simulink model "carry_skip_adder"  (R2022b)
settings: Solver=FixedStepDiscrete  StartTime=0.0  StopTime=10.0  RelTol=1e-3
PreLoadFcn:
  | addpath('C:\Course_Material\UofT\ECE1718\assignment2\matlab_tests\hdlimport\carry_skip_adder');
libraries: simulink x240, hdlsllib x97
(part 2 of 2)

== system carry_skip_adder/carry_skip_adder/adder_4bit/full_adder03 ==
  a : Inport  OutDataTypeStr=fixdt(0, 1, 0)  SampleTime=-1
  b : Inport  Port=2  OutDataTypeStr=fixdt(0, 1, 0)  SampleTime=-1
  c_in : Inport  Port=3  OutDataTypeStr=fixdt(0, 1, 0)  SampleTime=-1
  Bit_AND : simulink/Logic and Bit Operations/Bitwise Operator  logicop=AND  UseBitMask=off  NumInputPorts=2  BitMask=double(0)  BitMaskRealWorld=Real World Value
  Bit_AND_1 : simulink/Logic and Bit Operations/Bitwise Operator  logicop=AND  UseBitMask=off  NumInputPorts=2  BitMask=double(0)  BitMaskRealWorld=Real World Value
  Bit_OR : simulink/Logic and Bit Operations/Bitwise Operator  logicop=OR  UseBitMask=off  NumInputPorts=2  BitMask=double(0)  BitMaskRealWorld=Real World Value
  Bit_XOR : simulink/Logic and Bit Operations/Bitwise Operator  logicop=XOR  UseBitMask=off  NumInputPorts=2  BitMask=double(0)  BitMaskRealWorld=Real World Value
  Bit_XOR_1 : simulink/Logic and Bit Operations/Bitwise Operator  logicop=XOR  UseBitMask=off  NumInputPorts=2  BitMask=double(0)  BitMaskRealWorld=Real World Value
  Bit_XOR_2 : simulink/Logic and Bit Operations/Bitwise Operator  logicop=XOR  UseBitMask=off  NumInputPorts=2  BitMask=double(0)  BitMaskRealWorld=Real World Value
  sum : Outport  OutDataTypeStr=fixdt(0, 1, 0)  SampleTime=-1
  c_out : Outport  Port=2  OutDataTypeStr=fixdt(0, 1, 0)  SampleTime=-1
  wires:
  a/1 -> Bit_AND_1/1, Bit_XOR_2/1, Bit_XOR_1/1
  b/1 -> Bit_AND_1/2, Bit_XOR_2/2, Bit_XOR_1/2
  Bit_AND/1 -> Bit_OR/1
  Bit_XOR/1 -> sum/1
  Bit_AND_1/1 -> Bit_OR/2
  Bit_XOR_2/1 -> Bit_AND/1
  Bit_XOR_1/1 -> Bit_XOR/1
  c_in/1 -> Bit_AND/2, Bit_XOR/2
  Bit_OR/1 -> c_out/1

== system carry_skip_adder/carry_skip_adder/adder_4bit1/full_adder0 ==
  a : Inport  OutDataTypeStr=fixdt(0, 1, 0)  SampleTime=-1
  b : Inport  Port=2  OutDataTypeStr=fixdt(0, 1, 0)  SampleTime=-1
  c_in : Inport  Port=3  OutDataTypeStr=fixdt(0, 1, 0)  SampleTime=-1
  Bit_AND : simulink/Logic and Bit Operations/Bitwise Operator  logicop=AND  UseBitMask=off  NumInputPorts=2  BitMask=double(0)  BitMaskRealWorld=Real World Value
  Bit_AND_1 : simulink/Logic and Bit Operations/Bitwise Operator  logicop=AND  UseBitMask=off  NumInputPorts=2  BitMask=double(0)  BitMaskRealWorld=Real World Value
  Bit_OR : simulink/Logic and Bit Operations/Bitwise Operator  logicop=OR  UseBitMask=off  NumInputPorts=2  BitMask=double(0)  BitMaskRealWorld=Real World Value
  Bit_XOR : simulink/Logic and Bit Operations/Bitwise Operator  logicop=XOR  UseBitMask=off  NumInputPorts=2  BitMask=double(0)  BitMaskRealWorld=Real World Value
  Bit_XOR_1 : simulink/Logic and Bit Operations/Bitwise Operator  logicop=XOR  UseBitMask=off  NumInputPorts=2  BitMask=double(0)  BitMaskRealWorld=Real World Value
  Bit_XOR_2 : simulink/Logic and Bit Operations/Bitwise Operator  logicop=XOR  UseBitMask=off  NumInputPorts=2  BitMask=double(0)  BitMaskRealWorld=Real World Value
  sum : Outport  OutDataTypeStr=fixdt(0, 1, 0)  SampleTime=-1
  c_out : Outport  Port=2  OutDataTypeStr=fixdt(0, 1, 0)  SampleTime=-1
  wires:
  a/1 -> Bit_AND_1/1, Bit_XOR_2/1, Bit_XOR_1/1
  Bit_XOR_1/1 -> Bit_XOR/1
  b/1 -> Bit_AND_1/2, Bit_XOR_2/2, Bit_XOR_1/2
  c_in/1 -> Bit_AND/2, Bit_XOR/2
  Bit_XOR/1 -> sum/1
  Bit_AND_1/1 -> Bit_OR/2
  Bit_XOR_2/1 -> Bit_AND/1
  Bit_AND/1 -> Bit_OR/1
  Bit_OR/1 -> c_out/1

== system carry_skip_adder/carry_skip_adder/adder_4bit1/full_adder01 ==
  a : Inport  OutDataTypeStr=fixdt(0, 1, 0)  SampleTime=-1
  b : Inport  Port=2  OutDataTypeStr=fixdt(0, 1, 0)  SampleTime=-1
  c_in : Inport  Port=3  OutDataTypeStr=fixdt(0, 1, 0)  SampleTime=-1
  Bit_AND : simulink/Logic and Bit Operations/Bitwise Operator  logicop=AND  UseBitMask=off  NumInputPorts=2  BitMask=double(0)  BitMaskRealWorld=Real World Value
  Bit_AND_1 : simulink/Logic and Bit Operations/Bitwise Operator  logicop=AND  UseBitMask=off  NumInputPorts=2  BitMask=double(0)  BitMaskRealWorld=Real World Value
  Bit_OR : simulink/Logic and Bit Operations/Bitwise Operator  logicop=OR  UseBitMask=off  NumInputPorts=2  BitMask=double(0)  BitMaskRealWorld=Real World Value
  Bit_XOR : simulink/Logic and Bit Operations/Bitwise Operator  logicop=XOR  UseBitMask=off  NumInputPorts=2  BitMask=double(0)  BitMaskRealWorld=Real World Value
  Bit_XOR_1 : simulink/Logic and Bit Operations/Bitwise Operator  logicop=XOR  UseBitMask=off  NumInputPorts=2  BitMask=double(0)  BitMaskRealWorld=Real World Value
  Bit_XOR_2 : simulink/Logic and Bit Operations/Bitwise Operator  logicop=XOR  UseBitMask=off  NumInputPorts=2  BitMask=double(0)  BitMaskRealWorld=Real World Value
  sum : Outport  OutDataTypeStr=fixdt(0, 1, 0)  SampleTime=-1
  c_out : Outport  Port=2  OutDataTypeStr=fixdt(0, 1, 0)  SampleTime=-1
  wires:
  a/1 -> Bit_AND_1/1, Bit_XOR_2/1, Bit_XOR_1/1
  Bit_AND/1 -> Bit_OR/1
  b/1 -> Bit_AND_1/2, Bit_XOR_1/2, Bit_XOR_2/2
  Bit_AND_1/1 -> Bit_OR/2
  Bit_XOR_1/1 -> Bit_XOR/1
  c_in/1 -> Bit_AND/2, Bit_XOR/2
  Bit_XOR/1 -> sum/1
  Bit_XOR_2/1 -> Bit_AND/1
  Bit_OR/1 -> c_out/1

== system carry_skip_adder/carry_skip_adder/adder_4bit1/full_adder02 ==
  a : Inport  OutDataTypeStr=fixdt(0, 1, 0)  SampleTime=-1
  b : Inport  Port=2  OutDataTypeStr=fixdt(0, 1, 0)  SampleTime=-1
  c_in : Inport  Port=3  OutDataTypeStr=fixdt(0, 1, 0)  SampleTime=-1
  Bit_AND : simulink/Logic and Bit Operations/Bitwise Operator  logicop=AND  UseBitMask=off  NumInputPorts=2  BitMask=double(0)  BitMaskRealWorld=Real World Value
  Bit_AND_1 : simulink/Logic and Bit Operations/Bitwise Operator  logicop=AND  UseBitMask=off  NumInputPorts=2  BitMask=double(0)  BitMaskRealWorld=Real World Value
  Bit_OR : simulink/Logic and Bit Operations/Bitwise Operator  logicop=OR  UseBitMask=off  NumInputPorts=2  BitMask=double(0)  BitMaskRealWorld=Real World Value
  Bit_XOR : simulink/Logic and Bit Operations/Bitwise Operator  logicop=XOR  UseBitMask=off  NumInputPorts=2  BitMask=double(0)  BitMaskRealWorld=Real World Value
  Bit_XOR_1 : simulink/Logic and Bit Operations/Bitwise Operator  logicop=XOR  UseBitMask=off  NumInputPorts=2  BitMask=double(0)  BitMaskRealWorld=Real World Value
  Bit_XOR_2 : simulink/Logic and Bit Operations/Bitwise Operator  logicop=XOR  UseBitMask=off  NumInputPorts=2  BitMask=double(0)  BitMaskRealWorld=Real World Value
  sum : Outport  OutDataTypeStr=fixdt(0, 1, 0)  SampleTime=-1
  c_out : Outport  Port=2  OutDataTypeStr=fixdt(0, 1, 0)  SampleTime=-1
  wires:
  a/1 -> Bit_AND_1/1, Bit_XOR_2/1, Bit_XOR_1/1
  b/1 -> Bit_AND_1/2, Bit_XOR_2/2, Bit_XOR_1/2
  Bit_AND_1/1 -> Bit_OR/2
  Bit_XOR_1/1 -> Bit_XOR/1
  c_in/1 -> Bit_XOR/2, Bit_AND/2
  Bit_XOR/1 -> sum/1
  Bit_XOR_2/1 -> Bit_AND/1
  Bit_AND/1 -> Bit_OR/1
  Bit_OR/1 -> c_out/1

== system carry_skip_adder/carry_skip_adder/adder_4bit1/full_adder03 ==
  a : Inport  OutDataTypeStr=fixdt(0, 1, 0)  SampleTime=-1
  b : Inport  Port=2  OutDataTypeStr=fixdt(0, 1, 0)  SampleTime=-1
  c_in : Inport  Port=3  OutDataTypeStr=fixdt(0, 1, 0)  SampleTime=-1
  Bit_AND : simulink/Logic and Bit Operations/Bitwise Operator  logicop=AND  UseBitMask=off  NumInputPorts=2  BitMask=double(0)  BitMaskRealWorld=Real World Value
  Bit_AND_1 : simulink/Logic and Bit Operations/Bitwise Operator  logicop=AND  UseBitMask=off  NumInputPorts=2  BitMask=double(0)  BitMaskRealWorld=Real World Value
  Bit_OR : simulink/Logic and Bit Operations/Bitwise Operator  logicop=OR  UseBitMask=off  NumInputPorts=2  BitMask=double(0)  BitMaskRealWorld=Real World Value
  Bit_XOR : simulink/Logic and Bit Operations/Bitwise Operator  logicop=XOR  UseBitMask=off  NumInputPorts=2  BitMask=double(0)  BitMaskRealWorld=Real World Value
  Bit_XOR_1 : simulink/Logic and Bit Operations/Bitwise Operator  logicop=XOR  UseBitMask=off  NumInputPorts=2  BitMask=double(0)  BitMaskRealWorld=Real World Value
  Bit_XOR_2 : simulink/Logic and Bit Operations/Bitwise Operator  logicop=XOR  UseBitMask=off  NumInputPorts=2  BitMask=double(0)  BitMaskRealWorld=Real World Value
  sum : Outport  OutDataTypeStr=fixdt(0, 1, 0)  SampleTime=-1
  c_out : Outport  Port=2  OutDataTypeStr=fixdt(0, 1, 0)  SampleTime=-1
  wires:
  Bit_XOR/1 -> sum/1
  Bit_XOR_2/1 -> Bit_AND/1
  a/1 -> Bit_AND_1/1, Bit_XOR_2/1, Bit_XOR_1/1
  Bit_AND/1 -> Bit_OR/1
  Bit_AND_1/1 -> Bit_OR/2
  b/1 -> Bit_AND_1/2, Bit_XOR_2/2, Bit_XOR_1/2
  Bit_XOR_1/1 -> Bit_XOR/1
  c_in/1 -> Bit_AND/2, Bit_XOR/2
  Bit_OR/1 -> c_out/1

== system carry_skip_adder/carry_skip_adder/adder_4bit2/full_adder0 ==
  a : Inport  OutDataTypeStr=fixdt(0, 1, 0)  SampleTime=-1
  b : Inport  Port=2  OutDataTypeStr=fixdt(0, 1, 0)  SampleTime=-1
  c_in : Inport  Port=3  OutDataTypeStr=fixdt(0, 1, 0)  SampleTime=-1
  Bit_AND : simulink/Logic and Bit Operations/Bitwise Operator  logicop=AND  UseBitMask=off  NumInputPorts=2  BitMask=double(0)  BitMaskRealWorld=Real World Value
  Bit_AND_1 : simulink/Logic and Bit Operations/Bitwise Operator  logicop=AND  UseBitMask=off  NumInputPorts=2  BitMask=double(0)  BitMaskRealWorld=Real World Value
  Bit_OR : simulink/Logic and Bit Operations/Bitwise Operator  logicop=OR  UseBitMask=off  NumInputPorts=2  BitMask=double(0)  BitMaskRealWorld=Real World Value
  Bit_XOR : simulink/Logic and Bit Operations/Bitwise Operator  logicop=XOR  UseBitMask=off  NumInputPorts=2  BitMask=double(0)  BitMaskRealWorld=Real World Value
  Bit_XOR_1 : simulink/Logic and Bit Operations/Bitwise Operator  logicop=XOR  UseBitMask=off  NumInputPorts=2  BitMask=double(0)  BitMaskRealWorld=Real World Value
  Bit_XOR_2 : simulink/Logic and Bit Operations/Bitwise Operator  logicop=XOR  UseBitMask=off  NumInputPorts=2  BitMask=double(0)  BitMaskRealWorld=Real World Value
  sum : Outport  OutDataTypeStr=fixdt(0, 1, 0)  SampleTime=-1
  c_out : Outport  Port=2  OutDataTypeStr=fixdt(0, 1, 0)  SampleTime=-1
  wires:
  a/1 -> Bit_XOR_2/1, Bit_AND_1/1, Bit_XOR_1/1
  Bit_XOR_1/1 -> Bit_XOR/1
  b/1 -> Bit_XOR_2/2, Bit_AND_1/2, Bit_XOR_1/2
  Bit_XOR/1 -> sum/1
  c_in/1 -> Bit_AND/2, Bit_XOR/2
  Bit_XOR_2/1 -> Bit_AND/1
  Bit_AND_1/1 -> Bit_OR/2
  Bit_AND/1 -> Bit_OR/1
  Bit_OR/1 -> c_out/1

== system carry_skip_adder/carry_skip_adder/adder_4bit2/full_adder01 ==
  a : Inport  OutDataTypeStr=fixdt(0, 1, 0)  SampleTime=-1
  b : Inport  Port=2  OutDataTypeStr=fixdt(0, 1, 0)  SampleTime=-1
  c_in : Inport  Port=3  OutDataTypeStr=fixdt(0, 1, 0)  SampleTime=-1
  Bit_AND : simulink/Logic and Bit Operations/Bitwise Operator  logicop=AND  UseBitMask=off  NumInputPorts=2  BitMask=double(0)  BitMaskRealWorld=Real World Value
  Bit_AND_1 : simulink/Logic and Bit Operations/Bitwise Operator  logicop=AND  UseBitMask=off  NumInputPorts=2  BitMask=double(0)  BitMaskRealWorld=Real World Value
  Bit_OR : simulink/Logic and Bit Operations/Bitwise Operator  logicop=OR  UseBitMask=off  NumInputPorts=2  BitMask=double(0)  BitMaskRealWorld=Real World Value
  Bit_XOR : simulink/Logic and Bit Operations/Bitwise Operator  logicop=XOR  UseBitMask=off  NumInputPorts=2  BitMask=double(0)  BitMaskRealWorld=Real World Value
  Bit_XOR_1 : simulink/Logic and Bit Operations/Bitwise Operator  logicop=XOR  UseBitMask=off  NumInputPorts=2  BitMask=double(0)  BitMaskRealWorld=Real World Value
  Bit_XOR_2 : simulink/Logic and Bit Operations/Bitwise Operator  logicop=XOR  UseBitMask=off  NumInputPorts=2  BitMask=double(0)  BitMaskRealWorld=Real World Value
  sum : Outport  OutDataTypeStr=fixdt(0, 1, 0)  SampleTime=-1
  c_out : Outport  Port=2  OutDataTypeStr=fixdt(0, 1, 0)  SampleTime=-1
  wires:
  a/1 -> Bit_AND_1/1, Bit_XOR_2/1, Bit_XOR_1/1
  Bit_AND/1 -> Bit_OR/1
  b/1 -> Bit_XOR_2/2, Bit_XOR_1/2, Bit_AND_1/2
  Bit_AND_1/1 -> Bit_OR/2
  Bit_XOR_1/1 -> Bit_XOR/1
  c_in/1 -> Bit_AND/2, Bit_XOR/2
  Bit_XOR/1 -> sum/1
  Bit_XOR_2/1 -> Bit_AND/1
  Bit_OR/1 -> c_out/1

== system carry_skip_adder/carry_skip_adder/adder_4bit2/full_adder02 ==
  a : Inport  OutDataTypeStr=fixdt(0, 1, 0)  SampleTime=-1
  b : Inport  Port=2  OutDataTypeStr=fixdt(0, 1, 0)  SampleTime=-1
  c_in : Inport  Port=3  OutDataTypeStr=fixdt(0, 1, 0)  SampleTime=-1
  Bit_AND : simulink/Logic and Bit Operations/Bitwise Operator  logicop=AND  UseBitMask=off  NumInputPorts=2  BitMask=double(0)  BitMaskRealWorld=Real World Value
  Bit_AND_1 : simulink/Logic and Bit Operations/Bitwise Operator  logicop=AND  UseBitMask=off  NumInputPorts=2  BitMask=double(0)  BitMaskRealWorld=Real World Value
  Bit_OR : simulink/Logic and Bit Operations/Bitwise Operator  logicop=OR  UseBitMask=off  NumInputPorts=2  BitMask=double(0)  BitMaskRealWorld=Real World Value
  Bit_XOR : simulink/Logic and Bit Operations/Bitwise Operator  logicop=XOR  UseBitMask=off  NumInputPorts=2  BitMask=double(0)  BitMaskRealWorld=Real World Value
  Bit_XOR_1 : simulink/Logic and Bit Operations/Bitwise Operator  logicop=XOR  UseBitMask=off  NumInputPorts=2  BitMask=double(0)  BitMaskRealWorld=Real World Value
  Bit_XOR_2 : simulink/Logic and Bit Operations/Bitwise Operator  logicop=XOR  UseBitMask=off  NumInputPorts=2  BitMask=double(0)  BitMaskRealWorld=Real World Value
  sum : Outport  OutDataTypeStr=fixdt(0, 1, 0)  SampleTime=-1
  c_out : Outport  Port=2  OutDataTypeStr=fixdt(0, 1, 0)  SampleTime=-1
  wires:
  a/1 -> Bit_AND_1/1, Bit_XOR_2/1, Bit_XOR_1/1
  b/1 -> Bit_AND_1/2, Bit_XOR_2/2, Bit_XOR_1/2
  Bit_AND_1/1 -> Bit_OR/2
  Bit_XOR_1/1 -> Bit_XOR/1
  c_in/1 -> Bit_AND/2, Bit_XOR/2
  Bit_XOR/1 -> sum/1
  Bit_XOR_2/1 -> Bit_AND/1
  Bit_AND/1 -> Bit_OR/1
  Bit_OR/1 -> c_out/1

== system carry_skip_adder/carry_skip_adder/adder_4bit2/full_adder03 ==
  a : Inport  OutDataTypeStr=fixdt(0, 1, 0)  SampleTime=-1
  b : Inport  Port=2  OutDataTypeStr=fixdt(0, 1, 0)  SampleTime=-1
  c_in : Inport  Port=3  OutDataTypeStr=fixdt(0, 1, 0)  SampleTime=-1
  Bit_AND : simulink/Logic and Bit Operations/Bitwise Operator  logicop=AND  UseBitMask=off  NumInputPorts=2  BitMask=double(0)  BitMaskRealWorld=Real World Value
  Bit_AND_1 : simulink/Logic and Bit Operations/Bitwise Operator  logicop=AND  UseBitMask=off  NumInputPorts=2  BitMask=double(0)  BitMaskRealWorld=Real World Value
  Bit_OR : simulink/Logic and Bit Operations/Bitwise Operator  logicop=OR  UseBitMask=off  NumInputPorts=2  BitMask=double(0)  BitMaskRealWorld=Real World Value
  Bit_XOR : simulink/Logic and Bit Operations/Bitwise Operator  logicop=XOR  UseBitMask=off  NumInputPorts=2  BitMask=double(0)  BitMaskRealWorld=Real World Value
  Bit_XOR_1 : simulink/Logic and Bit Operations/Bitwise Operator  logicop=XOR  UseBitMask=off  NumInputPorts=2  BitMask=double(0)  BitMaskRealWorld=Real World Value
  Bit_XOR_2 : simulink/Logic and Bit Operations/Bitwise Operator  logicop=XOR  UseBitMask=off  NumInputPorts=2  BitMask=double(0)  BitMaskRealWorld=Real World Value
  sum : Outport  OutDataTypeStr=fixdt(0, 1, 0)  SampleTime=-1
  c_out : Outport  Port=2  OutDataTypeStr=fixdt(0, 1, 0)  SampleTime=-1
  wires:
  a/1 -> Bit_AND_1/1, Bit_XOR_2/1, Bit_XOR_1/1
  Bit_AND/1 -> Bit_OR/1
  b/1 -> Bit_XOR_2/2, Bit_XOR_1/2, Bit_AND_1/2
  Bit_AND_1/1 -> Bit_OR/2
  Bit_XOR_1/1 -> Bit_XOR/1
  c_in/1 -> Bit_AND/2, Bit_XOR/2
  Bit_XOR/1 -> sum/1
  Bit_XOR_2/1 -> Bit_AND/1
  Bit_OR/1 -> c_out/1

== system carry_skip_adder/carry_skip_adder/adder_4bit3/full_adder0 ==
  a : Inport  OutDataTypeStr=fixdt(0, 1, 0)  SampleTime=-1
  b : Inport  Port=2  OutDataTypeStr=fixdt(0, 1, 0)  SampleTime=-1
  c_in : Inport  Port=3  OutDataTypeStr=fixdt(0, 1, 0)  SampleTime=-1
  Bit_AND : simulink/Logic and Bit Operations/Bitwise Operator  logicop=AND  UseBitMask=off  NumInputPorts=2  BitMask=double(0)  BitMaskRealWorld=Real World Value
  Bit_AND_1 : simulink/Logic and Bit Operations/Bitwise Operator  logicop=AND  UseBitMask=off  NumInputPorts=2  BitMask=double(0)  BitMaskRealWorld=Real World Value
  Bit_OR : simulink/Logic and Bit Operations/Bitwise Operator  logicop=OR  UseBitMask=off  NumInputPorts=2  BitMask=double(0)  BitMaskRealWorld=Real World Value
  Bit_XOR : simulink/Logic and Bit Operations/Bitwise Operator  logicop=XOR  UseBitMask=off  NumInputPorts=2  BitMask=double(0)  BitMaskRealWorld=Real World Value
  Bit_XOR_1 : simulink/Logic and Bit Operations/Bitwise Operator  logicop=XOR  UseBitMask=off  NumInputPorts=2  BitMask=double(0)  BitMaskRealWorld=Real World Value
  Bit_XOR_2 : simulink/Logic and Bit Operations/Bitwise Operator  logicop=XOR  UseBitMask=off  NumInputPorts=2  BitMask=double(0)  BitMaskRealWorld=Real World Value
  sum : Outport  OutDataTypeStr=fixdt(0, 1, 0)  SampleTime=-1
  c_out : Outport  Port=2  OutDataTypeStr=fixdt(0, 1, 0)  SampleTime=-1
  wires:
  Bit_AND_1/1 -> Bit_OR/2
  a/1 -> Bit_AND_1/1, Bit_XOR_2/1, Bit_XOR_1/1
  Bit_XOR_1/1 -> Bit_XOR/1
  b/1 -> Bit_AND_1/2, Bit_XOR_2/2, Bit_XOR_1/2
  c_in/1 -> Bit_AND/2, Bit_XOR/2
  Bit_XOR/1 -> sum/1
  Bit_XOR_2/1 -> Bit_AND/1
  Bit_AND/1 -> Bit_OR/1
  Bit_OR/1 -> c_out/1

== system carry_skip_adder/carry_skip_adder/adder_4bit3/full_adder01 ==
  a : Inport  OutDataTypeStr=fixdt(0, 1, 0)  SampleTime=-1
  b : Inport  Port=2  OutDataTypeStr=fixdt(0, 1, 0)  SampleTime=-1
  c_in : Inport  Port=3  OutDataTypeStr=fixdt(0, 1, 0)  SampleTime=-1
  Bit_AND : simulink/Logic and Bit Operations/Bitwise Operator  logicop=AND  UseBitMask=off  NumInputPorts=2  BitMask=double(0)  BitMaskRealWorld=Real World Value
  Bit_AND_1 : simulink/Logic and Bit Operations/Bitwise Operator  logicop=AND  UseBitMask=off  NumInputPorts=2  BitMask=double(0)  BitMaskRealWorld=Real World Value
  Bit_OR : simulink/Logic and Bit Operations/Bitwise Operator  logicop=OR  UseBitMask=off  NumInputPorts=2  BitMask=double(0)  BitMaskRealWorld=Real World Value
  Bit_XOR : simulink/Logic and Bit Operations/Bitwise Operator  logicop=XOR  UseBitMask=off  NumInputPorts=2  BitMask=double(0)  BitMaskRealWorld=Real World Value
  Bit_XOR_1 : simulink/Logic and Bit Operations/Bitwise Operator  logicop=XOR  UseBitMask=off  NumInputPorts=2  BitMask=double(0)  BitMaskRealWorld=Real World Value
  Bit_XOR_2 : simulink/Logic and Bit Operations/Bitwise Operator  logicop=XOR  UseBitMask=off  NumInputPorts=2  BitMask=double(0)  BitMaskRealWorld=Real World Value
  sum : Outport  OutDataTypeStr=fixdt(0, 1, 0)  SampleTime=-1
  c_out : Outport  Port=2  OutDataTypeStr=fixdt(0, 1, 0)  SampleTime=-1
  wires:
  a/1 -> Bit_AND_1/1, Bit_XOR_1/1, Bit_XOR_2/1
  Bit_AND/1 -> Bit_OR/1
  b/1 -> Bit_AND_1/2, Bit_XOR_2/2, Bit_XOR_1/2
  Bit_AND_1/1 -> Bit_OR/2
  Bit_XOR_1/1 -> Bit_XOR/1
  c_in/1 -> Bit_AND/2, Bit_XOR/2
  Bit_XOR/1 -> sum/1
  Bit_XOR_2/1 -> Bit_AND/1
  Bit_OR/1 -> c_out/1

== system carry_skip_adder/carry_skip_adder/adder_4bit3/full_adder02 ==
  a : Inport  OutDataTypeStr=fixdt(0, 1, 0)  SampleTime=-1
  b : Inport  Port=2  OutDataTypeStr=fixdt(0, 1, 0)  SampleTime=-1
  c_in : Inport  Port=3  OutDataTypeStr=fixdt(0, 1, 0)  SampleTime=-1
  Bit_AND : simulink/Logic and Bit Operations/Bitwise Operator  logicop=AND  UseBitMask=off  NumInputPorts=2  BitMask=double(0)  BitMaskRealWorld=Real World Value
  Bit_AND_1 : simulink/Logic and Bit Operations/Bitwise Operator  logicop=AND  UseBitMask=off  NumInputPorts=2  BitMask=double(0)  BitMaskRealWorld=Real World Value
  Bit_OR : simulink/Logic and Bit Operations/Bitwise Operator  logicop=OR  UseBitMask=off  NumInputPorts=2  BitMask=double(0)  BitMaskRealWorld=Real World Value
  Bit_XOR : simulink/Logic and Bit Operations/Bitwise Operator  logicop=XOR  UseBitMask=off  NumInputPorts=2  BitMask=double(0)  BitMaskRealWorld=Real World Value
  Bit_XOR_1 : simulink/Logic and Bit Operations/Bitwise Operator  logicop=XOR  UseBitMask=off  NumInputPorts=2  BitMask=double(0)  BitMaskRealWorld=Real World Value
  Bit_XOR_2 : simulink/Logic and Bit Operations/Bitwise Operator  logicop=XOR  UseBitMask=off  NumInputPorts=2  BitMask=double(0)  BitMaskRealWorld=Real World Value
  sum : Outport  OutDataTypeStr=fixdt(0, 1, 0)  SampleTime=-1
  c_out : Outport  Port=2  OutDataTypeStr=fixdt(0, 1, 0)  SampleTime=-1
  wires:
  a/1 -> Bit_AND_1/1, Bit_XOR_1/1, Bit_XOR_2/1
  b/1 -> Bit_AND_1/2, Bit_XOR_2/2, Bit_XOR_1/2
  Bit_AND_1/1 -> Bit_OR/2
  Bit_XOR_1/1 -> Bit_XOR/1
  c_in/1 -> Bit_AND/2, Bit_XOR/2
  Bit_XOR/1 -> sum/1
  Bit_XOR_2/1 -> Bit_AND/1
  Bit_AND/1 -> Bit_OR/1
  Bit_OR/1 -> c_out/1

== system carry_skip_adder/carry_skip_adder/adder_4bit3/full_adder03 ==
  a : Inport  OutDataTypeStr=fixdt(0, 1, 0)  SampleTime=-1
  b : Inport  Port=2  OutDataTypeStr=fixdt(0, 1, 0)  SampleTime=-1
  c_in : Inport  Port=3  OutDataTypeStr=fixdt(0, 1, 0)  SampleTime=-1
  Bit_AND : simulink/Logic and Bit Operations/Bitwise Operator  logicop=AND  UseBitMask=off  NumInputPorts=2  BitMask=double(0)  BitMaskRealWorld=Real World Value
  Bit_AND_1 : simulink/Logic and Bit Operations/Bitwise Operator  logicop=AND  UseBitMask=off  NumInputPorts=2  BitMask=double(0)  BitMaskRealWorld=Real World Value
  Bit_OR : simulink/Logic and Bit Operations/Bitwise Operator  logicop=OR  UseBitMask=off  NumInputPorts=2  BitMask=double(0)  BitMaskRealWorld=Real World Value
  Bit_XOR : simulink/Logic and Bit Operations/Bitwise Operator  logicop=XOR  UseBitMask=off  NumInputPorts=2  BitMask=double(0)  BitMaskRealWorld=Real World Value
  Bit_XOR_1 : simulink/Logic and Bit Operations/Bitwise Operator  logicop=XOR  UseBitMask=off  NumInputPorts=2  BitMask=double(0)  BitMaskRealWorld=Real World Value
  Bit_XOR_2 : simulink/Logic and Bit Operations/Bitwise Operator  logicop=XOR  UseBitMask=off  NumInputPorts=2  BitMask=double(0)  BitMaskRealWorld=Real World Value
  sum : Outport  OutDataTypeStr=fixdt(0, 1, 0)  SampleTime=-1
  c_out : Outport  Port=2  OutDataTypeStr=fixdt(0, 1, 0)  SampleTime=-1
  wires:
  a/1 -> Bit_AND_1/1, Bit_XOR_2/1, Bit_XOR_1/1
  Bit_AND/1 -> Bit_OR/1
  b/1 -> Bit_AND_1/2, Bit_XOR_1/2, Bit_XOR_2/2
  Bit_AND_1/1 -> Bit_OR/2
  Bit_XOR_1/1 -> Bit_XOR/1
  c_in/1 -> Bit_AND/2, Bit_XOR/2
  Bit_XOR/1 -> sum/1
  Bit_XOR_2/1 -> Bit_AND/1
  Bit_OR/1 -> c_out/1

== system carry_skip_adder/carry_skip_adder/adder_4bit4/full_adder0 ==
  a : Inport  OutDataTypeStr=fixdt(0, 1, 0)  SampleTime=-1
  b : Inport  Port=2  OutDataTypeStr=fixdt(0, 1, 0)  SampleTime=-1
  c_in : Inport  Port=3  OutDataTypeStr=fixdt(0, 1, 0)  SampleTime=-1
  Bit_AND : simulink/Logic and Bit Operations/Bitwise Operator  logicop=AND  UseBitMask=off  NumInputPorts=2  BitMask=double(0)  BitMaskRealWorld=Real World Value
  Bit_AND_1 : simulink/Logic and Bit Operations/Bitwise Operator  logicop=AND  UseBitMask=off  NumInputPorts=2  BitMask=double(0)  BitMaskRealWorld=Real World Value
  Bit_OR : simulink/Logic and Bit Operations/Bitwise Operator  logicop=OR  UseBitMask=off  NumInputPorts=2  BitMask=double(0)  BitMaskRealWorld=Real World Value
  Bit_XOR : simulink/Logic and Bit Operations/Bitwise Operator  logicop=XOR  UseBitMask=off  NumInputPorts=2  BitMask=double(0)  BitMaskRealWorld=Real World Value
  Bit_XOR_1 : simulink/Logic and Bit Operations/Bitwise Operator  logicop=XOR  UseBitMask=off  NumInputPorts=2  BitMask=double(0)  BitMaskRealWorld=Real World Value
  Bit_XOR_2 : simulink/Logic and Bit Operations/Bitwise Operator  logicop=XOR  UseBitMask=off  NumInputPorts=2  BitMask=double(0)  BitMaskRealWorld=Real World Value
  sum : Outport  OutDataTypeStr=fixdt(0, 1, 0)  SampleTime=-1
  c_out : Outport  Port=2  OutDataTypeStr=fixdt(0, 1, 0)  SampleTime=-1
  wires:
  a/1 -> Bit_XOR_2/1, Bit_XOR_1/1, Bit_AND_1/1
  Bit_XOR_1/1 -> Bit_XOR/1
  b/1 -> Bit_AND_1/2, Bit_XOR_2/2, Bit_XOR_1/2
  c_in/1 -> Bit_AND/2, Bit_XOR/2
  Bit_XOR/1 -> sum/1
  Bit_AND_1/1 -> Bit_OR/2
  Bit_XOR_2/1 -> Bit_AND/1
  Bit_AND/1 -> Bit_OR/1
  Bit_OR/1 -> c_out/1

== system carry_skip_adder/carry_skip_adder/adder_4bit4/full_adder01 ==
  a : Inport  OutDataTypeStr=fixdt(0, 1, 0)  SampleTime=-1
  b : Inport  Port=2  OutDataTypeStr=fixdt(0, 1, 0)  SampleTime=-1
  c_in : Inport  Port=3  OutDataTypeStr=fixdt(0, 1, 0)  SampleTime=-1
  Bit_AND : simulink/Logic and Bit Operations/Bitwise Operator  logicop=AND  UseBitMask=off  NumInputPorts=2  BitMask=double(0)  BitMaskRealWorld=Real World Value
  Bit_AND_1 : simulink/Logic and Bit Operations/Bitwise Operator  logicop=AND  UseBitMask=off  NumInputPorts=2  BitMask=double(0)  BitMaskRealWorld=Real World Value
  Bit_OR : simulink/Logic and Bit Operations/Bitwise Operator  logicop=OR  UseBitMask=off  NumInputPorts=2  BitMask=double(0)  BitMaskRealWorld=Real World Value
  Bit_XOR : simulink/Logic and Bit Operations/Bitwise Operator  logicop=XOR  UseBitMask=off  NumInputPorts=2  BitMask=double(0)  BitMaskRealWorld=Real World Value
  Bit_XOR_1 : simulink/Logic and Bit Operations/Bitwise Operator  logicop=XOR  UseBitMask=off  NumInputPorts=2  BitMask=double(0)  BitMaskRealWorld=Real World Value
  Bit_XOR_2 : simulink/Logic and Bit Operations/Bitwise Operator  logicop=XOR  UseBitMask=off  NumInputPorts=2  BitMask=double(0)  BitMaskRealWorld=Real World Value
  sum : Outport  OutDataTypeStr=fixdt(0, 1, 0)  SampleTime=-1
  c_out : Outport  Port=2  OutDataTypeStr=fixdt(0, 1, 0)  SampleTime=-1
  wires:
  a/1 -> Bit_XOR_2/1, Bit_AND_1/1, Bit_XOR_1/1
  Bit_AND/1 -> Bit_OR/1
  b/1 -> Bit_XOR_2/2, Bit_XOR_1/2, Bit_AND_1/2
  Bit_AND_1/1 -> Bit_OR/2
  Bit_XOR_1/1 -> Bit_XOR/1
  c_in/1 -> Bit_AND/2, Bit_XOR/2
  Bit_XOR/1 -> sum/1
  Bit_XOR_2/1 -> Bit_AND/1
  Bit_OR/1 -> c_out/1

== system carry_skip_adder/carry_skip_adder/adder_4bit4/full_adder02 ==
  a : Inport  OutDataTypeStr=fixdt(0, 1, 0)  SampleTime=-1
  b : Inport  Port=2  OutDataTypeStr=fixdt(0, 1, 0)  SampleTime=-1
  c_in : Inport  Port=3  OutDataTypeStr=fixdt(0, 1, 0)  SampleTime=-1
  Bit_AND : simulink/Logic and Bit Operations/Bitwise Operator  logicop=AND  UseBitMask=off  NumInputPorts=2  BitMask=double(0)  BitMaskRealWorld=Real World Value
  Bit_AND_1 : simulink/Logic and Bit Operations/Bitwise Operator  logicop=AND  UseBitMask=off  NumInputPorts=2  BitMask=double(0)  BitMaskRealWorld=Real World Value
  Bit_OR : simulink/Logic and Bit Operations/Bitwise Operator  logicop=OR  UseBitMask=off  NumInputPorts=2  BitMask=double(0)  BitMaskRealWorld=Real World Value
  Bit_XOR : simulink/Logic and Bit Operations/Bitwise Operator  logicop=XOR  UseBitMask=off  NumInputPorts=2  BitMask=double(0)  BitMaskRealWorld=Real World Value
  Bit_XOR_1 : simulink/Logic and Bit Operations/Bitwise Operator  logicop=XOR  UseBitMask=off  NumInputPorts=2  BitMask=double(0)  BitMaskRealWorld=Real World Value
  Bit_XOR_2 : simulink/Logic and Bit Operations/Bitwise Operator  logicop=XOR  UseBitMask=off  NumInputPorts=2  BitMask=double(0)  BitMaskRealWorld=Real World Value
  sum : Outport  OutDataTypeStr=fixdt(0, 1, 0)  SampleTime=-1
  c_out : Outport  Port=2  OutDataTypeStr=fixdt(0, 1, 0)  SampleTime=-1
  wires:
  a/1 -> Bit_AND_1/1, Bit_XOR_2/1, Bit_XOR_1/1
  b/1 -> Bit_XOR_2/2, Bit_XOR_1/2, Bit_AND_1/2
  Bit_AND_1/1 -> Bit_OR/2
  Bit_XOR_1/1 -> Bit_XOR/1
  c_in/1 -> Bit_AND/2, Bit_XOR/2
  Bit_XOR/1 -> sum/1
  Bit_XOR_2/1 -> Bit_AND/1
  Bit_AND/1 -> Bit_OR/1
  Bit_OR/1 -> c_out/1

== system carry_skip_adder/carry_skip_adder/adder_4bit4/full_adder03 ==
  a : Inport  OutDataTypeStr=fixdt(0, 1, 0)  SampleTime=-1
  b : Inport  Port=2  OutDataTypeStr=fixdt(0, 1, 0)  SampleTime=-1
  c_in : Inport  Port=3  OutDataTypeStr=fixdt(0, 1, 0)  SampleTime=-1
  Bit_AND : simulink/Logic and Bit Operations/Bitwise Operator  logicop=AND  UseBitMask=off  NumInputPorts=2  BitMask=double(0)  BitMaskRealWorld=Real World Value
  Bit_AND_1 : simulink/Logic and Bit Operations/Bitwise Operator  logicop=AND  UseBitMask=off  NumInputPorts=2  BitMask=double(0)  BitMaskRealWorld=Real World Value
  Bit_OR : simulink/Logic and Bit Operations/Bitwise Operator  logicop=OR  UseBitMask=off  NumInputPorts=2  BitMask=double(0)  BitMaskRealWorld=Real World Value
  Bit_XOR : simulink/Logic and Bit Operations/Bitwise Operator  logicop=XOR  UseBitMask=off  NumInputPorts=2  BitMask=double(0)  BitMaskRealWorld=Real World Value
  Bit_XOR_1 : simulink/Logic and Bit Operations/Bitwise Operator  logicop=XOR  UseBitMask=off  NumInputPorts=2  BitMask=double(0)  BitMaskRealWorld=Real World Value
  Bit_XOR_2 : simulink/Logic and Bit Operations/Bitwise Operator  logicop=XOR  UseBitMask=off  NumInputPorts=2  BitMask=double(0)  BitMaskRealWorld=Real World Value
  sum : Outport  OutDataTypeStr=fixdt(0, 1, 0)  SampleTime=-1
  c_out : Outport  Port=2  OutDataTypeStr=fixdt(0, 1, 0)  SampleTime=-1
  wires:
  a/1 -> Bit_AND_1/1, Bit_XOR_2/1, Bit_XOR_1/1
  Bit_AND/1 -> Bit_OR/1
  b/1 -> Bit_AND_1/2, Bit_XOR_2/2, Bit_XOR_1/2
  Bit_AND_1/1 -> Bit_OR/2
  Bit_XOR_1/1 -> Bit_XOR/1
  c_in/1 -> Bit_AND/2, Bit_XOR/2
  Bit_XOR/1 -> sum/1
  Bit_XOR_2/1 -> Bit_AND/1
  Bit_OR/1 -> c_out/1

== system carry_skip_adder/carry_skip_adder/adder_4bit5/full_adder0 ==
  a : Inport  OutDataTypeStr=fixdt(0, 1, 0)  SampleTime=-1
  b : Inport  Port=2  OutDataTypeStr=fixdt(0, 1, 0)  SampleTime=-1
  c_in : Inport  Port=3  OutDataTypeStr=fixdt(0, 1, 0)  SampleTime=-1
  Bit_AND : simulink/Logic and Bit Operations/Bitwise Operator  logicop=AND  UseBitMask=off  NumInputPorts=2  BitMask=double(0)  BitMaskRealWorld=Real World Value
  Bit_AND_1 : simulink/Logic and Bit Operations/Bitwise Operator  logicop=AND  UseBitMask=off  NumInputPorts=2  BitMask=double(0)  BitMaskRealWorld=Real World Value
  Bit_OR : simulink/Logic and Bit Operations/Bitwise Operator  logicop=OR  UseBitMask=off  NumInputPorts=2  BitMask=double(0)  BitMaskRealWorld=Real World Value
  Bit_XOR : simulink/Logic and Bit Operations/Bitwise Operator  logicop=XOR  UseBitMask=off  NumInputPorts=2  BitMask=double(0)  BitMaskRealWorld=Real World Value
  Bit_XOR_1 : simulink/Logic and Bit Operations/Bitwise Operator  logicop=XOR  UseBitMask=off  NumInputPorts=2  BitMask=double(0)  BitMaskRealWorld=Real World Value
  Bit_XOR_2 : simulink/Logic and Bit Operations/Bitwise Operator  logicop=XOR  UseBitMask=off  NumInputPorts=2  BitMask=double(0)  BitMaskRealWorld=Real World Value
  sum : Outport  OutDataTypeStr=fixdt(0, 1, 0)  SampleTime=-1
  c_out : Outport  Port=2  OutDataTypeStr=fixdt(0, 1, 0)  SampleTime=-1
  wires:
  a/1 -> Bit_AND_1/1, Bit_XOR_2/1, Bit_XOR_1/1
  Bit_XOR_1/1 -> Bit_XOR/1
  b/1 -> Bit_XOR_2/2, Bit_XOR_1/2, Bit_AND_1/2
  c_in/1 -> Bit_AND/2, Bit_XOR/2
  Bit_XOR/1 -> sum/1
  Bit_XOR_2/1 -> Bit_AND/1
  Bit_AND_1/1 -> Bit_OR/2
  Bit_AND/1 -> Bit_OR/1
  Bit_OR/1 -> c_out/1

== system carry_skip_adder/carry_skip_adder/adder_4bit5/full_adder01 ==
  a : Inport  OutDataTypeStr=fixdt(0, 1, 0)  SampleTime=-1
  b : Inport  Port=2  OutDataTypeStr=fixdt(0, 1, 0)  SampleTime=-1
  c_in : Inport  Port=3  OutDataTypeStr=fixdt(0, 1, 0)  SampleTime=-1
  Bit_AND : simulink/Logic and Bit Operations/Bitwise Operator  logicop=AND  UseBitMask=off  NumInputPorts=2  BitMask=double(0)  BitMaskRealWorld=Real World Value
  Bit_AND_1 : simulink/Logic and Bit Operations/Bitwise Operator  logicop=AND  UseBitMask=off  NumInputPorts=2  BitMask=double(0)  BitMaskRealWorld=Real World Value
  Bit_OR : simulink/Logic and Bit Operations/Bitwise Operator  logicop=OR  UseBitMask=off  NumInputPorts=2  BitMask=double(0)  BitMaskRealWorld=Real World Value
  Bit_XOR : simulink/Logic and Bit Operations/Bitwise Operator  logicop=XOR  UseBitMask=off  NumInputPorts=2  BitMask=double(0)  BitMaskRealWorld=Real World Value
  Bit_XOR_1 : simulink/Logic and Bit Operations/Bitwise Operator  logicop=XOR  UseBitMask=off  NumInputPorts=2  BitMask=double(0)  BitMaskRealWorld=Real World Value
  Bit_XOR_2 : simulink/Logic and Bit Operations/Bitwise Operator  logicop=XOR  UseBitMask=off  NumInputPorts=2  BitMask=double(0)  BitMaskRealWorld=Real World Value
  sum : Outport  OutDataTypeStr=fixdt(0, 1, 0)  SampleTime=-1
  c_out : Outport  Port=2  OutDataTypeStr=fixdt(0, 1, 0)  SampleTime=-1
  wires:
  a/1 -> Bit_AND_1/1, Bit_XOR_2/1, Bit_XOR_1/1
  Bit_AND/1 -> Bit_OR/1
  b/1 -> Bit_AND_1/2, Bit_XOR_2/2, Bit_XOR_1/2
  Bit_AND_1/1 -> Bit_OR/2
  Bit_XOR_1/1 -> Bit_XOR/1
  c_in/1 -> Bit_AND/2, Bit_XOR/2
  Bit_XOR/1 -> sum/1
  Bit_XOR_2/1 -> Bit_AND/1
  Bit_OR/1 -> c_out/1

== system carry_skip_adder/carry_skip_adder/adder_4bit5/full_adder02 ==
  a : Inport  OutDataTypeStr=fixdt(0, 1, 0)  SampleTime=-1
  b : Inport  Port=2  OutDataTypeStr=fixdt(0, 1, 0)  SampleTime=-1
  c_in : Inport  Port=3  OutDataTypeStr=fixdt(0, 1, 0)  SampleTime=-1
  Bit_AND : simulink/Logic and Bit Operations/Bitwise Operator  logicop=AND  UseBitMask=off  NumInputPorts=2  BitMask=double(0)  BitMaskRealWorld=Real World Value
  Bit_AND_1 : simulink/Logic and Bit Operations/Bitwise Operator  logicop=AND  UseBitMask=off  NumInputPorts=2  BitMask=double(0)  BitMaskRealWorld=Real World Value
  Bit_OR : simulink/Logic and Bit Operations/Bitwise Operator  logicop=OR  UseBitMask=off  NumInputPorts=2  BitMask=double(0)  BitMaskRealWorld=Real World Value
  Bit_XOR : simulink/Logic and Bit Operations/Bitwise Operator  logicop=XOR  UseBitMask=off  NumInputPorts=2  BitMask=double(0)  BitMaskRealWorld=Real World Value
  Bit_XOR_1 : simulink/Logic and Bit Operations/Bitwise Operator  logicop=XOR  UseBitMask=off  NumInputPorts=2  BitMask=double(0)  BitMaskRealWorld=Real World Value
  Bit_XOR_2 : simulink/Logic and Bit Operations/Bitwise Operator  logicop=XOR  UseBitMask=off  NumInputPorts=2  BitMask=double(0)  BitMaskRealWorld=Real World Value
  sum : Outport  OutDataTypeStr=fixdt(0, 1, 0)  SampleTime=-1
  c_out : Outport  Port=2  OutDataTypeStr=fixdt(0, 1, 0)  SampleTime=-1
  wires:
  a/1 -> Bit_AND_1/1, Bit_XOR_2/1, Bit_XOR_1/1
  b/1 -> Bit_XOR_2/2, Bit_XOR_1/2, Bit_AND_1/2
  Bit_AND_1/1 -> Bit_OR/2
  Bit_XOR_1/1 -> Bit_XOR/1
  c_in/1 -> Bit_AND/2, Bit_XOR/2
  Bit_XOR/1 -> sum/1
  Bit_XOR_2/1 -> Bit_AND/1
  Bit_AND/1 -> Bit_OR/1
  Bit_OR/1 -> c_out/1

== system carry_skip_adder/carry_skip_adder/adder_4bit5/full_adder03 ==
  a : Inport  OutDataTypeStr=fixdt(0, 1, 0)  SampleTime=-1
  b : Inport  Port=2  OutDataTypeStr=fixdt(0, 1, 0)  SampleTime=-1
  c_in : Inport  Port=3  OutDataTypeStr=fixdt(0, 1, 0)  SampleTime=-1
  Bit_AND : simulink/Logic and Bit Operations/Bitwise Operator  logicop=AND  UseBitMask=off  NumInputPorts=2  BitMask=double(0)  BitMaskRealWorld=Real World Value
  Bit_AND_1 : simulink/Logic and Bit Operations/Bitwise Operator  logicop=AND  UseBitMask=off  NumInputPorts=2  BitMask=double(0)  BitMaskRealWorld=Real World Value
  Bit_OR : simulink/Logic and Bit Operations/Bitwise Operator  logicop=OR  UseBitMask=off  NumInputPorts=2  BitMask=double(0)  BitMaskRealWorld=Real World Value
  Bit_XOR : simulink/Logic and Bit Operations/Bitwise Operator  logicop=XOR  UseBitMask=off  NumInputPorts=2  BitMask=double(0)  BitMaskRealWorld=Real World Value
  Bit_XOR_1 : simulink/Logic and Bit Operations/Bitwise Operator  logicop=XOR  UseBitMask=off  NumInputPorts=2  BitMask=double(0)  BitMaskRealWorld=Real World Value
  Bit_XOR_2 : simulink/Logic and Bit Operations/Bitwise Operator  logicop=XOR  UseBitMask=off  NumInputPorts=2  BitMask=double(0)  BitMaskRealWorld=Real World Value
  sum : Outport  OutDataTypeStr=fixdt(0, 1, 0)  SampleTime=-1
  c_out : Outport  Port=2  OutDataTypeStr=fixdt(0, 1, 0)  SampleTime=-1
  wires:
  a/1 -> Bit_AND_1/1, Bit_XOR_2/1, Bit_XOR_1/1
  b/1 -> Bit_AND_1/2, Bit_XOR_2/2, Bit_XOR_1/2
  Bit_AND_1/1 -> Bit_OR/2
  Bit_XOR_1/1 -> Bit_XOR/1
  c_in/1 -> Bit_AND/2, Bit_XOR/2
  Bit_AND/1 -> Bit_OR/1
  Bit_XOR_2/1 -> Bit_AND/1
  Bit_XOR/1 -> sum/1
  Bit_OR/1 -> c_out/1

== system carry_skip_adder/carry_skip_adder/adder_4bit6/full_adder0 ==
  a : Inport  OutDataTypeStr=fixdt(0, 1, 0)  SampleTime=-1
  b : Inport  Port=2  OutDataTypeStr=fixdt(0, 1, 0)  SampleTime=-1
  c_in : Inport  Port=3  OutDataTypeStr=fixdt(0, 1, 0)  SampleTime=-1
  Bit_AND : simulink/Logic and Bit Operations/Bitwise Operator  logicop=AND  UseBitMask=off  NumInputPorts=2  BitMask=double(0)  BitMaskRealWorld=Real World Value
  Bit_AND_1 : simulink/Logic and Bit Operations/Bitwise Operator  logicop=AND  UseBitMask=off  NumInputPorts=2  BitMask=double(0)  BitMaskRealWorld=Real World Value
  Bit_OR : simulink/Logic and Bit Operations/Bitwise Operator  logicop=OR  UseBitMask=off  NumInputPorts=2  BitMask=double(0)  BitMaskRealWorld=Real World Value
  Bit_XOR : simulink/Logic and Bit Operations/Bitwise Operator  logicop=XOR  UseBitMask=off  NumInputPorts=2  BitMask=double(0)  BitMaskRealWorld=Real World Value
  Bit_XOR_1 : simulink/Logic and Bit Operations/Bitwise Operator  logicop=XOR  UseBitMask=off  NumInputPorts=2  BitMask=double(0)  BitMaskRealWorld=Real World Value
  Bit_XOR_2 : simulink/Logic and Bit Operations/Bitwise Operator  logicop=XOR  UseBitMask=off  NumInputPorts=2  BitMask=double(0)  BitMaskRealWorld=Real World Value
  sum : Outport  OutDataTypeStr=fixdt(0, 1, 0)  SampleTime=-1
  c_out : Outport  Port=2  OutDataTypeStr=fixdt(0, 1, 0)  SampleTime=-1
  wires:
  a/1 -> Bit_AND_1/1, Bit_XOR_2/1, Bit_XOR_1/1
  Bit_XOR_1/1 -> Bit_XOR/1
  b/1 -> Bit_AND_1/2, Bit_XOR_2/2, Bit_XOR_1/2
  c_in/1 -> Bit_AND/2, Bit_XOR/2
  Bit_XOR/1 -> sum/1
  Bit_XOR_2/1 -> Bit_AND/1
  Bit_AND_1/1 -> Bit_OR/2
  Bit_AND/1 -> Bit_OR/1
  Bit_OR/1 -> c_out/1

== system carry_skip_adder/carry_skip_adder/adder_4bit6/full_adder01 ==
  a : Inport  OutDataTypeStr=fixdt(0, 1, 0)  SampleTime=-1
  b : Inport  Port=2  OutDataTypeStr=fixdt(0, 1, 0)  SampleTime=-1
  c_in : Inport  Port=3  OutDataTypeStr=fixdt(0, 1, 0)  SampleTime=-1
  Bit_AND : simulink/Logic and Bit Operations/Bitwise Operator  logicop=AND  UseBitMask=off  NumInputPorts=2  BitMask=double(0)  BitMaskRealWorld=Real World Value
  Bit_AND_1 : simulink/Logic and Bit Operations/Bitwise Operator  logicop=AND  UseBitMask=off  NumInputPorts=2  BitMask=double(0)  BitMaskRealWorld=Real World Value
  Bit_OR : simulink/Logic and Bit Operations/Bitwise Operator  logicop=OR  UseBitMask=off  NumInputPorts=2  BitMask=double(0)  BitMaskRealWorld=Real World Value
  Bit_XOR : simulink/Logic and Bit Operations/Bitwise Operator  logicop=XOR  UseBitMask=off  NumInputPorts=2  BitMask=double(0)  BitMaskRealWorld=Real World Value
  Bit_XOR_1 : simulink/Logic and Bit Operations/Bitwise Operator  logicop=XOR  UseBitMask=off  NumInputPorts=2  BitMask=double(0)  BitMaskRealWorld=Real World Value
  Bit_XOR_2 : simulink/Logic and Bit Operations/Bitwise Operator  logicop=XOR  UseBitMask=off  NumInputPorts=2  BitMask=double(0)  BitMaskRealWorld=Real World Value
  sum : Outport  OutDataTypeStr=fixdt(0, 1, 0)  SampleTime=-1
  c_out : Outport  Port=2  OutDataTypeStr=fixdt(0, 1, 0)  SampleTime=-1
  wires:
  Bit_XOR/1 -> sum/1
  Bit_XOR_2/1 -> Bit_AND/1
  a/1 -> Bit_AND_1/1, Bit_XOR_2/1, Bit_XOR_1/1
  Bit_AND/1 -> Bit_OR/1
  b/1 -> Bit_AND_1/2, Bit_XOR_1/2, Bit_XOR_2/2
  Bit_AND_1/1 -> Bit_OR/2
  Bit_XOR_1/1 -> Bit_XOR/1
  c_in/1 -> Bit_XOR/2, Bit_AND/2
  Bit_OR/1 -> c_out/1

== system carry_skip_adder/carry_skip_adder/adder_4bit6/full_adder02 ==
  a : Inport  OutDataTypeStr=fixdt(0, 1, 0)  SampleTime=-1
  b : Inport  Port=2  OutDataTypeStr=fixdt(0, 1, 0)  SampleTime=-1
  c_in : Inport  Port=3  OutDataTypeStr=fixdt(0, 1, 0)  SampleTime=-1
  Bit_AND : simulink/Logic and Bit Operations/Bitwise Operator  logicop=AND  UseBitMask=off  NumInputPorts=2  BitMask=double(0)  BitMaskRealWorld=Real World Value
  Bit_AND_1 : simulink/Logic and Bit Operations/Bitwise Operator  logicop=AND  UseBitMask=off  NumInputPorts=2  BitMask=double(0)  BitMaskRealWorld=Real World Value
  Bit_OR : simulink/Logic and Bit Operations/Bitwise Operator  logicop=OR  UseBitMask=off  NumInputPorts=2  BitMask=double(0)  BitMaskRealWorld=Real World Value
  Bit_XOR : simulink/Logic and Bit Operations/Bitwise Operator  logicop=XOR  UseBitMask=off  NumInputPorts=2  BitMask=double(0)  BitMaskRealWorld=Real World Value
  Bit_XOR_1 : simulink/Logic and Bit Operations/Bitwise Operator  logicop=XOR  UseBitMask=off  NumInputPorts=2  BitMask=double(0)  BitMaskRealWorld=Real World Value
  Bit_XOR_2 : simulink/Logic and Bit Operations/Bitwise Operator  logicop=XOR  UseBitMask=off  NumInputPorts=2  BitMask=double(0)  BitMaskRealWorld=Real World Value
  sum : Outport  OutDataTypeStr=fixdt(0, 1, 0)  SampleTime=-1
  c_out : Outport  Port=2  OutDataTypeStr=fixdt(0, 1, 0)  SampleTime=-1
  wires:
  a/1 -> Bit_AND_1/1, Bit_XOR_2/1, Bit_XOR_1/1
  b/1 -> Bit_AND_1/2, Bit_XOR_2/2, Bit_XOR_1/2
  Bit_AND_1/1 -> Bit_OR/2
  Bit_XOR_1/1 -> Bit_XOR/1
  c_in/1 -> Bit_AND/2, Bit_XOR/2
  Bit_XOR/1 -> sum/1
  Bit_XOR_2/1 -> Bit_AND/1
  Bit_AND/1 -> Bit_OR/1
  Bit_OR/1 -> c_out/1

== system carry_skip_adder/carry_skip_adder/adder_4bit6/full_adder03 ==
  a : Inport  OutDataTypeStr=fixdt(0, 1, 0)  SampleTime=-1
  b : Inport  Port=2  OutDataTypeStr=fixdt(0, 1, 0)  SampleTime=-1
  c_in : Inport  Port=3  OutDataTypeStr=fixdt(0, 1, 0)  SampleTime=-1
  Bit_AND : simulink/Logic and Bit Operations/Bitwise Operator  logicop=AND  UseBitMask=off  NumInputPorts=2  BitMask=double(0)  BitMaskRealWorld=Real World Value
  Bit_AND_1 : simulink/Logic and Bit Operations/Bitwise Operator  logicop=AND  UseBitMask=off  NumInputPorts=2  BitMask=double(0)  BitMaskRealWorld=Real World Value
  Bit_OR : simulink/Logic and Bit Operations/Bitwise Operator  logicop=OR  UseBitMask=off  NumInputPorts=2  BitMask=double(0)  BitMaskRealWorld=Real World Value
  Bit_XOR : simulink/Logic and Bit Operations/Bitwise Operator  logicop=XOR  UseBitMask=off  NumInputPorts=2  BitMask=double(0)  BitMaskRealWorld=Real World Value
  Bit_XOR_1 : simulink/Logic and Bit Operations/Bitwise Operator  logicop=XOR  UseBitMask=off  NumInputPorts=2  BitMask=double(0)  BitMaskRealWorld=Real World Value
  Bit_XOR_2 : simulink/Logic and Bit Operations/Bitwise Operator  logicop=XOR  UseBitMask=off  NumInputPorts=2  BitMask=double(0)  BitMaskRealWorld=Real World Value
  sum : Outport  OutDataTypeStr=fixdt(0, 1, 0)  SampleTime=-1
  c_out : Outport  Port=2  OutDataTypeStr=fixdt(0, 1, 0)  SampleTime=-1
  wires:
  a/1 -> Bit_AND_1/1, Bit_XOR_1/1, Bit_XOR_2/1
  Bit_AND/1 -> Bit_OR/1
  b/1 -> Bit_XOR_2/2, Bit_AND_1/2, Bit_XOR_1/2
  Bit_AND_1/1 -> Bit_OR/2
  Bit_XOR_1/1 -> Bit_XOR/1
  c_in/1 -> Bit_XOR/2, Bit_AND/2
  Bit_XOR/1 -> sum/1
  Bit_XOR_2/1 -> Bit_AND/1
  Bit_OR/1 -> c_out/1

== system carry_skip_adder/carry_skip_adder/adder_4bit7/full_adder0 ==
  a : Inport  OutDataTypeStr=fixdt(0, 1, 0)  SampleTime=-1
  b : Inport  Port=2  OutDataTypeStr=fixdt(0, 1, 0)  SampleTime=-1
  c_in : Inport  Port=3  OutDataTypeStr=fixdt(0, 1, 0)  SampleTime=-1
  Bit_AND : simulink/Logic and Bit Operations/Bitwise Operator  logicop=AND  UseBitMask=off  NumInputPorts=2  BitMask=double(0)  BitMaskRealWorld=Real World Value
  Bit_AND_1 : simulink/Logic and Bit Operations/Bitwise Operator  logicop=AND  UseBitMask=off  NumInputPorts=2  BitMask=double(0)  BitMaskRealWorld=Real World Value
  Bit_OR : simulink/Logic and Bit Operations/Bitwise Operator  logicop=OR  UseBitMask=off  NumInputPorts=2  BitMask=double(0)  BitMaskRealWorld=Real World Value
  Bit_XOR : simulink/Logic and Bit Operations/Bitwise Operator  logicop=XOR  UseBitMask=off  NumInputPorts=2  BitMask=double(0)  BitMaskRealWorld=Real World Value
  Bit_XOR_1 : simulink/Logic and Bit Operations/Bitwise Operator  logicop=XOR  UseBitMask=off  NumInputPorts=2  BitMask=double(0)  BitMaskRealWorld=Real World Value
  Bit_XOR_2 : simulink/Logic and Bit Operations/Bitwise Operator  logicop=XOR  UseBitMask=off  NumInputPorts=2  BitMask=double(0)  BitMaskRealWorld=Real World Value
  sum : Outport  OutDataTypeStr=fixdt(0, 1, 0)  SampleTime=-1
  c_out : Outport  Port=2  OutDataTypeStr=fixdt(0, 1, 0)  SampleTime=-1
  wires:
  a/1 -> Bit_AND_1/1, Bit_XOR_2/1, Bit_XOR_1/1
  Bit_XOR_1/1 -> Bit_XOR/1
  b/1 -> Bit_AND_1/2, Bit_XOR_2/2, Bit_XOR_1/2
  c_in/1 -> Bit_AND/2, Bit_XOR/2
  Bit_XOR/1 -> sum/1
  Bit_XOR_2/1 -> Bit_AND/1
  Bit_AND_1/1 -> Bit_OR/2
  Bit_AND/1 -> Bit_OR/1
  Bit_OR/1 -> c_out/1

== system carry_skip_adder/carry_skip_adder/adder_4bit7/full_adder01 ==
  a : Inport  OutDataTypeStr=fixdt(0, 1, 0)  SampleTime=-1
  b : Inport  Port=2  OutDataTypeStr=fixdt(0, 1, 0)  SampleTime=-1
  c_in : Inport  Port=3  OutDataTypeStr=fixdt(0, 1, 0)  SampleTime=-1
  Bit_AND : simulink/Logic and Bit Operations/Bitwise Operator  logicop=AND  UseBitMask=off  NumInputPorts=2  BitMask=double(0)  BitMaskRealWorld=Real World Value
  Bit_AND_1 : simulink/Logic and Bit Operations/Bitwise Operator  logicop=AND  UseBitMask=off  NumInputPorts=2  BitMask=double(0)  BitMaskRealWorld=Real World Value
  Bit_OR : simulink/Logic and Bit Operations/Bitwise Operator  logicop=OR  UseBitMask=off  NumInputPorts=2  BitMask=double(0)  BitMaskRealWorld=Real World Value
  Bit_XOR : simulink/Logic and Bit Operations/Bitwise Operator  logicop=XOR  UseBitMask=off  NumInputPorts=2  BitMask=double(0)  BitMaskRealWorld=Real World Value
  Bit_XOR_1 : simulink/Logic and Bit Operations/Bitwise Operator  logicop=XOR  UseBitMask=off  NumInputPorts=2  BitMask=double(0)  BitMaskRealWorld=Real World Value
  Bit_XOR_2 : simulink/Logic and Bit Operations/Bitwise Operator  logicop=XOR  UseBitMask=off  NumInputPorts=2  BitMask=double(0)  BitMaskRealWorld=Real World Value
  sum : Outport  OutDataTypeStr=fixdt(0, 1, 0)  SampleTime=-1
  c_out : Outport  Port=2  OutDataTypeStr=fixdt(0, 1, 0)  SampleTime=-1
  wires:
  Bit_XOR/1 -> sum/1
  Bit_XOR_2/1 -> Bit_AND/1
  a/1 -> Bit_XOR_2/1, Bit_AND_1/1, Bit_XOR_1/1
  Bit_AND/1 -> Bit_OR/1
  b/1 -> Bit_XOR_2/2, Bit_AND_1/2, Bit_XOR_1/2
  Bit_AND_1/1 -> Bit_OR/2
  Bit_XOR_1/1 -> Bit_XOR/1
  c_in/1 -> Bit_AND/2, Bit_XOR/2
  Bit_OR/1 -> c_out/1

== system carry_skip_adder/carry_skip_adder/adder_4bit7/full_adder02 ==
  a : Inport  OutDataTypeStr=fixdt(0, 1, 0)  SampleTime=-1
  b : Inport  Port=2  OutDataTypeStr=fixdt(0, 1, 0)  SampleTime=-1
  c_in : Inport  Port=3  OutDataTypeStr=fixdt(0, 1, 0)  SampleTime=-1
  Bit_AND : simulink/Logic and Bit Operations/Bitwise Operator  logicop=AND  UseBitMask=off  NumInputPorts=2  BitMask=double(0)  BitMaskRealWorld=Real World Value
  Bit_AND_1 : simulink/Logic and Bit Operations/Bitwise Operator  logicop=AND  UseBitMask=off  NumInputPorts=2  BitMask=double(0)  BitMaskRealWorld=Real World Value
  Bit_OR : simulink/Logic and Bit Operations/Bitwise Operator  logicop=OR  UseBitMask=off  NumInputPorts=2  BitMask=double(0)  BitMaskRealWorld=Real World Value
  Bit_XOR : simulink/Logic and Bit Operations/Bitwise Operator  logicop=XOR  UseBitMask=off  NumInputPorts=2  BitMask=double(0)  BitMaskRealWorld=Real World Value
  Bit_XOR_1 : simulink/Logic and Bit Operations/Bitwise Operator  logicop=XOR  UseBitMask=off  NumInputPorts=2  BitMask=double(0)  BitMaskRealWorld=Real World Value
  Bit_XOR_2 : simulink/Logic and Bit Operations/Bitwise Operator  logicop=XOR  UseBitMask=off  NumInputPorts=2  BitMask=double(0)  BitMaskRealWorld=Real World Value
  sum : Outport  OutDataTypeStr=fixdt(0, 1, 0)  SampleTime=-1
  c_out : Outport  Port=2  OutDataTypeStr=fixdt(0, 1, 0)  SampleTime=-1
  wires:
  a/1 -> Bit_AND_1/1, Bit_XOR_1/1, Bit_XOR_2/1
  Bit_XOR/1 -> sum/1
  Bit_XOR_2/1 -> Bit_AND/1
  b/1 -> Bit_AND_1/2, Bit_XOR_2/2, Bit_XOR_1/2
  Bit_AND_1/1 -> Bit_OR/2
  Bit_XOR_1/1 -> Bit_XOR/1
  c_in/1 -> Bit_AND/2, Bit_XOR/2
  Bit_AND/1 -> Bit_OR/1
  Bit_OR/1 -> c_out/1

== system carry_skip_adder/carry_skip_adder/adder_4bit7/full_adder03 ==
  a : Inport  OutDataTypeStr=fixdt(0, 1, 0)  SampleTime=-1
  b : Inport  Port=2  OutDataTypeStr=fixdt(0, 1, 0)  SampleTime=-1
  c_in : Inport  Port=3  OutDataTypeStr=fixdt(0, 1, 0)  SampleTime=-1
  Bit_AND : simulink/Logic and Bit Operations/Bitwise Operator  logicop=AND  UseBitMask=off  NumInputPorts=2  BitMask=double(0)  BitMaskRealWorld=Real World Value
  Bit_AND_1 : simulink/Logic and Bit Operations/Bitwise Operator  logicop=AND  UseBitMask=off  NumInputPorts=2  BitMask=double(0)  BitMaskRealWorld=Real World Value
  Bit_OR : simulink/Logic and Bit Operations/Bitwise Operator  logicop=OR  UseBitMask=off  NumInputPorts=2  BitMask=double(0)  BitMaskRealWorld=Real World Value
  Bit_XOR : simulink/Logic and Bit Operations/Bitwise Operator  logicop=XOR  UseBitMask=off  NumInputPorts=2  BitMask=double(0)  BitMaskRealWorld=Real World Value
  Bit_XOR_1 : simulink/Logic and Bit Operations/Bitwise Operator  logicop=XOR  UseBitMask=off  NumInputPorts=2  BitMask=double(0)  BitMaskRealWorld=Real World Value
  Bit_XOR_2 : simulink/Logic and Bit Operations/Bitwise Operator  logicop=XOR  UseBitMask=off  NumInputPorts=2  BitMask=double(0)  BitMaskRealWorld=Real World Value
  sum : Outport  OutDataTypeStr=fixdt(0, 1, 0)  SampleTime=-1
  c_out : Outport  Port=2  OutDataTypeStr=fixdt(0, 1, 0)  SampleTime=-1
  wires:
  a/1 -> Bit_AND_1/1, Bit_XOR_2/1, Bit_XOR_1/1
  Bit_AND/1 -> Bit_OR/1
  b/1 -> Bit_AND_1/2, Bit_XOR_2/2, Bit_XOR_1/2
  Bit_AND_1/1 -> Bit_OR/2
  Bit_XOR_1/1 -> Bit_XOR/1
  c_in/1 -> Bit_AND/2, Bit_XOR/2
  Bit_XOR/1 -> sum/1
  Bit_XOR_2/1 -> Bit_AND/1
  Bit_OR/1 -> c_out/1

== matlab function carry_skip_adder/MATLAB Function ==
  data: input input; output output
function output = fixed_point_to_int(input)
    temp = fi(input, 1, 32, 8);
    output = int32(temp * (2 ^ 8));
end

== matlab function carry_skip_adder/MATLAB Function2 ==
  data: input input; output output
function output = int_to_fixed_point(input)
    temp = double(input);
    output = fi(temp / (2 ^ 8), 1, 32, 8);
end

== matlab function carry_skip_adder/MATLAB Function3 ==
  data: input input; output output
function output = fixed_point_to_int(input)
    temp = fi(input, 1, 32, 8);
    output = int32(temp * (2 ^ 8));
end

== matlab function carry_skip_adder/MATLAB Function4 ==
  data: input input; output output
function output = fixed_point_to_int(input)
    temp = fi(input, 1, 32, 8);
    output = int32(temp * (2 ^ 8));
end

== matlab function carry_skip_adder/MATLAB Function5 ==
  data: input input; output output
function output = int_to_fixed_point(input)
    temp = double(input);
    output = fi(temp / (2 ^ 8), 1, 32, 8);
end

== matlab function carry_skip_adder/MATLAB Function1 ==
  data: input input; output output
function output = fixed_point_to_int(input)
    temp = fi(input, 1, 32, 8);
    output = int32(temp * (2 ^ 8));
end
